simulink subsystem "Day6_Scenario_1"  (R2024a)
settings: Solver=VariableStepAuto  StartTime=0.0  StopTime=10.0  RelTol=1e-3
undefined symbols (not defined in the file): route1_waypoint, route2_waypoint, route3_waypoint
libraries: CarMaker4SL x15
settings Model: Creator=junhyung.cha  LastModifiedBy=User

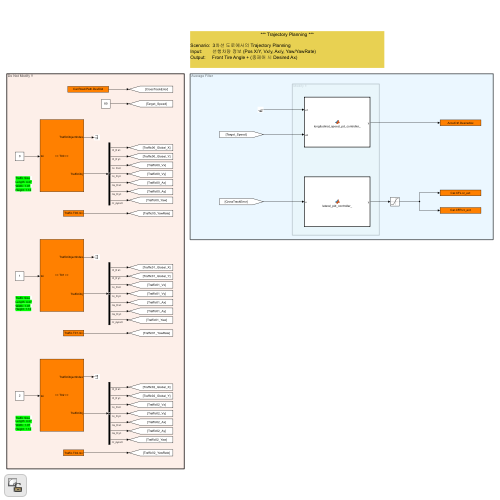
[thumbnail: Simulink's stored preview of the top-level diagram]
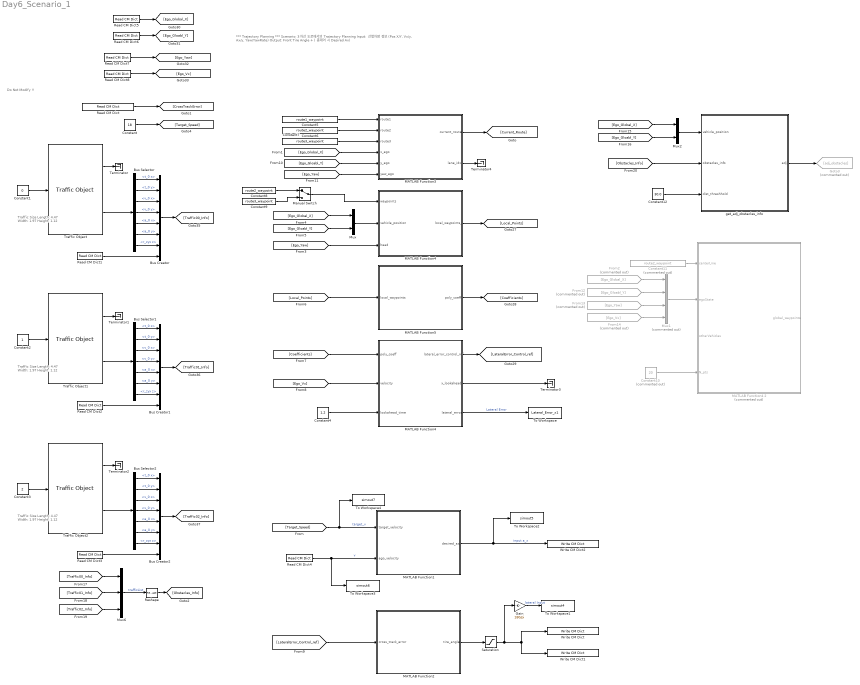
== system Day6_Scenario_1 ==
  note: Do Not Modify !!
  note: Traffic Size
      | Length: 4.47
      | Width: 1.97
      | Height: 1.12
  note: Traffic Size
      | Length: 4.47
      | Width: 1.97
      | Height: 1.12
  note: Traffic Size
      | Length: 4.47
      | Width: 1.97
      | Height: 1.12
  note: *** Trajectory Planning ***
      |
      | Scenario: 3차선 도로에서의 Trajectory Planning
      | Input: 선행차량 정보 (Pos X/Y, Vx/y, Ax/y, Yaw/YawRate)
      | Output: Front Tire Angle + (종제어 시 Desired Ax)
  Bus Creator : BusCreator  Inputs=8
  Bus Creator1 : BusCreator  Inputs=8
  Bus Creator2 : BusCreator  Inputs=8
  Bus Selector : BusSelector  OutputSignals=t_0 x,t_0 y,v_0 x,v_0 y,a_0 x,a_0 y,r_zyx z
  Bus Selector1 : BusSelector  OutputSignals=t_0 x,t_0 y,v_0 x,v_0 y,a_0 x,a_0 y,r_zyx z
  Bus Selector2 : BusSelector  OutputSignals=t_0 x,t_0 y,v_0 x,v_0 y,a_0 x,a_0 y,r_zyx z
  Constant : Constant  Value=18
  Constant1 : Constant  Value=0
  Constant10 : Constant  Commented=on  Value=20
  Constant11 : Constant  Commented=on  Value=route2_waypoint  SampleTime=-1
  Constant12 : Constant  Value=30.0
  Constant2 : Constant
  Constant3 : Constant  Value=2
  Constant4 : Constant  Value=1.2
  Constant5 : Constant  Value=route1_waypoint  SampleTime=-1
  Constant6 : Constant  Value=route2_waypoint  SampleTime=-1
  Constant7 : Constant  Value=route3_waypoint
  Constant8 : Constant  Value=route2_waypoint  SampleTime=-1
  Constant9 : Constant  Value=route3_waypoint
  From12 : From  Commented=on  GotoTag=Ego_Gloabl_Y
  From13 : From  Commented=on  GotoTag=Ego_Yaw
  From14 : From  Commented=on  GotoTag=Ego_Vx
  From2 : From  Commented=on  GotoTag=Ego_Global_X
  Gain : Gain  Gain=180/pi
  Goto3 : Goto  Commented=on  GotoTag=adj_obstacles
  MATLAB Function1 : MATLAB Function  TreatAsAtomicUnit=on
  MATLAB Function2 : MATLAB Function  TreatAsAtomicUnit=on
  MATLAB Function3 : MATLAB Function  TreatAsAtomicUnit=on
  MATLAB Function4 : MATLAB Function  TreatAsAtomicUnit=on
  "MATLAB Function4 " : MATLAB Function  TreatAsAtomicUnit=on
  MATLAB Function4 2 : MATLAB Function  Commented=on  TreatAsAtomicUnit=on
  MATLAB Function5 : MATLAB Function  TreatAsAtomicUnit=on
  Manual Switch : ManualSwitch  varsize=on
  Mux : Mux  Inputs=2
  Mux1 : Mux  Commented=on
  Mux2 : Mux  Inputs=2
  Mux6 : Mux  Inputs=3
  Read CM Dict : CarMaker4SL/Read CM Dict  xname=Car.Road.Path.DevDist  xsync=off  xstime=Inherited
  Read CM Dict1 : CarMaker4SL/Read CM Dict  xname=Traffic.T00.rzv  xsync=off  xstime=Inherited
  Read CM Dict2 : CarMaker4SL/Read CM Dict  xname=Traffic.T01.rzv  xsync=off  xstime=Inherited
  Read CM Dict3 : CarMaker4SL/Read CM Dict  xname=Traffic.T02.rzv  xsync=off  xstime=Inherited
  Read CM Dict4 : CarMaker4SL/Read CM Dict  xname=Car.v  xsync=off  xstime=Inherited
  Read CM Dict5 : CarMaker4SL/Read CM Dict  xname=Car.Fr1.tx  xsync=off  xstime=Inherited
  Read CM Dict6 : CarMaker4SL/Read CM Dict  xname=Car.Fr1.ty  xsync=off  xstime=Inherited
  Read CM Dict7 : CarMaker4SL/Read CM Dict  xname=Car.Fr1.rz  xsync=off  xstime=Inherited
  Read CM Dict8 : CarMaker4SL/Read CM Dict  xname=Car.v  xsync=off  xstime=Inherited
  Reshape : Reshape  OutputDimensionality=Customize  OutputDimensions=[3, 8]
  Saturation : Saturate  UpperLimit=2  LowerLimit=-2
  Terminator{,1..4} (5 alike) : Terminator
  To Workspace : ToWorkspace  VariableName=Lateral_Error_x1  SaveFormat=Timeseries  SampleTime=-1
  To Workspace1 : ToWorkspace  VariableName=simout4  SaveFormat=Timeseries  SampleTime=-1
  To Workspace2 : ToWorkspace  VariableName=simout5  SaveFormat=Timeseries  SampleTime=-1
  To Workspace3 : ToWorkspace  VariableName=simout6  SaveFormat=Timeseries  SampleTime=-1
  To Workspace4 : ToWorkspace  VariableName=simout7  SaveFormat=Timeseries  SampleTime=-1
  Traffic Object : CarMaker4SL/Traffic Object  xname=T00  ximode=Traffic Id  xstime=Inherited
      settings: SourceProductName=CarMaker4SL
  Traffic Object1 : CarMaker4SL/Traffic Object  xname=T01  ximode=Traffic Id  xstime=Inherited
      settings: SourceProductName=CarMaker4SL
  Traffic Object2 : CarMaker4SL/Traffic Object  xname=T02  ximode=Traffic Id  xstime=Inherited
      settings: SourceProductName=CarMaker4SL
  Write CM Dict : CarMaker4SL/Write CM Dict  xname=Car.CFL.rz_ext  xsync=off
  Write CM Dict1 : CarMaker4SL/Write CM Dict  xname=Car.CFR.rz_ext  xsync=off
  Write CM Dict2 : CarMaker4SL/Write CM Dict  xname=AccelCtrl.DesiredAx  xsync=off
  get_adj_obstacles_info : MATLAB Function  TreatAsAtomicUnit=on
  wires:
  Saturation/1 -> Write CM Dict1/1, Write CM Dict/1, Gain/1
  Constant1/1 -> Traffic Object/1
  MATLAB Function2/1(tire_angle) -> Saturation/1
  MATLAB Function1/1(desired_ax) -> Write CM Dict2/1, To Workspace2/1  "input a_x"
  [LateralError_Control_ref] -> MATLAB Function2/1(cross_track_error)
  Read CM Dict/1 -> [CrossTrackError]
  Constant/1 -> [Target_Speed]
  Bus Selector/4 -> Bus Creator/4  "<v_0 y>"
  Traffic Object/1 -> Terminator/1
  Bus Selector/3 -> Bus Creator/3  "<v_0 x>"
  Traffic Object/2 -> Bus Selector/1
  Bus Selector/1 -> Bus Creator/1  "<t_0 x>"
  Bus Selector/2 -> Bus Creator/2  "<t_0 y>"
  Read CM Dict1/1 -> Bus Creator/8
  Bus Selector/5 -> Bus Creator/5  "<a_0 x>"
  Bus Selector/6 -> Bus Creator/6  "<a_0 y>"
  Bus Selector/7 -> Bus Creator/7  "<r_zyx z>"
  Read CM Dict2/1 -> Bus Creator1/8
  Bus Selector1/1 -> Bus Creator1/1  "<t_0 x>"
  Bus Selector1/5 -> Bus Creator1/5  "<a_0 x>"
  Bus Selector1/6 -> Bus Creator1/6  "<a_0 y>"
  Bus Selector1/7 -> Bus Creator1/7  "<r_zyx z>"
  Traffic Object1/1 -> Terminator1/1
  Bus Selector1/4 -> Bus Creator1/4  "<v_0 y>"
  Constant2/1 -> Traffic Object1/1
  Bus Selector1/3 -> Bus Creator1/3  "<v_0 x>"
  Bus Selector1/2 -> Bus Creator1/2  "<t_0 y>"
  Bus Selector2/3 -> Bus Creator2/3  "<v_0 x>"
  Bus Selector2/2 -> Bus Creator2/2  "<t_0 y>"
  Bus Selector2/1 -> Bus Creator2/1  "<t_0 x>"
  Bus Selector2/6 -> Bus Creator2/6  "<a_0 y>"
  Constant3/1 -> Traffic Object2/1
  Traffic Object2/1 -> Terminator2/1
  Bus Selector2/7 -> Bus Creator2/7  "<r_zyx z>"
  Bus Selector2/5 -> Bus Creator2/5  "<a_0 x>"
  Read CM Dict3/1 -> Bus Creator2/8
  Bus Selector2/4 -> Bus Creator2/4  "<v_0 y>"
  [Target_Speed] -> MATLAB Function1/1(target_velocity), To Workspace4/1  "target_v"
  Read CM Dict4/1 -> MATLAB Function1/2(ego_velocity), To Workspace3/1  "v"
  [Ego_Gloabl_Y] -> Mux/2
  [Ego_Yaw] -> "MATLAB Function4 "/3(head)
  "MATLAB Function4 "/1(local_waypoints_) -> [Local_Points]
  Mux/1 -> "MATLAB Function4 "/2(vehicle_position)
  [Ego_Global_X] -> Mux/1
  MATLAB Function4/3(lateral_error) -> To Workspace/1  "Lateral Error"
  Constant4/1 -> MATLAB Function4/3(lookahead_time)
  MATLAB Function4/2(x_lookahead) -> Terminator3/1
  [Local_Points] -> MATLAB Function5/1(local_waypoints)
  MATLAB Function4/1(lateral_error_control_ref) -> [LateralError_Control_ref]
  MATLAB Function5/1(poly_coeff) -> [Coefficients]
  [Coefficients] -> MATLAB Function4/1(poly_coeff)
  [Ego_Vx] -> MATLAB Function4/2(velocity)
  [Ego_Global_X] -> MATLAB Function3/4(x_ego)
  [Ego_Gloabl_Y] -> MATLAB Function3/5(y_ego)
  [Ego_Yaw] -> MATLAB Function3/6(yaw_ego)
  MATLAB Function3/1(current_route) -> [Current_Route]
  Constant5/1 -> MATLAB Function3/1(route1)
  Constant6/1 -> MATLAB Function3/2(route2)
  Constant7/1 -> MATLAB Function3/3(route3)
  Read CM Dict5/1 -> [Ego_Global_X]
  Read CM Dict6/1 -> [Ego_Gloabl_Y]
  Read CM Dict8/1 -> [Ego_Vx]
  Read CM Dict7/1 -> [Ego_Yaw]
  Gain/1 -> To Workspace1/1  "lateral Input"
  Constant8/1 -> Manual Switch/1
  Constant9/1 -> Manual Switch/2
  Manual Switch/1 -> "MATLAB Function4 "/1(waypoints)
  Traffic Object1/2 -> Bus Selector1/1
  Traffic Object2/2 -> Bus Selector2/1
  Constant10/1 -> MATLAB Function4 2/4(N_pts)
  Constant11/1 -> MATLAB Function4 2/1(centerLine)
  From12/1 -> Mux1/2
  From2/1 -> Mux1/1
  From13/1 -> Mux1/3
  From14/1 -> Mux1/4
  Mux1/1 -> MATLAB Function4 2/2(egoState)
  [Ego_Gloabl_Y] -> Mux2/2
  [Ego_Global_X] -> Mux2/1
  Mux2/1 -> get_adj_obstacles_info/1(vehicle_position)
  Bus Creator/1 -> [Traffic00_Info]
  Bus Creator1/1 -> [Traffic01_Info]
  Bus Creator2/1 -> [Traffic02_Info]
  [Traffic00_Info] -> Mux6/1
  [Traffic01_Info] -> Mux6/2
  [Traffic02_Info] -> Mux6/3
  Mux6/1 -> Reshape/1  "trafficList"
  MATLAB Function3/2(lane_idx) -> Terminator4/1
  get_adj_obstacles_info/1(adj) -> Goto3/1
  Reshape/1 -> [Obstacles_Info]
  Constant12/1 -> get_adj_obstacles_info/3(dist_threshhold)
  [Obstacles_Info] -> get_adj_obstacles_info/2(obstacles_info)

== matlab function Day6_Scenario_1/MATLAB Function1 ==
  settings: updateMethod=DISCRETE  sampleTime=0.1
  data: target_velocity input; desired_ax output; ego_velocity input
function desired_ax = longitudinal_speed_pi_controller_(target_velocity, ego_velocity)
    desired_ax = longitudinal_speed_pi_controller_mfile(target_velocity, ego_velocity);
end


function desired_ax = longitudinal_speed_pi_controller_mfile(target_velocity, ego_velocity)
     
    persistent error_sum
    dt = 0.1;
    
    error = target_velocity - ego_velocity;

    if isempty(error_sum)
        error_sum = 0;
    else
        error_sum = error_sum + error * dt;
    end

    Kp = 0.215;
    Ki = 0.001;

    P_term = Kp*error;
    I_term = Ki*error_sum;
    
    desired_ax = (P_term + I_term);

end

== matlab function Day6_Scenario_1/MATLAB Function2 ==
  settings: updateMethod=DISCRETE  sampleTime=0.05
  data: cross_track_error input; tire_angle output
function tire_angle = lateral_pid_controller_(cross_track_error)
    tire_angle = lateral_pid_controller_mfile(cross_track_error);
end

function tire_angle = lateral_pid_controller_mfile(cross_track_error)
    persistent error_prev error_sum
    % error = average_filter_mfile(cross_track_error);
    error = cross_track_error;
    
    dt = 0.05;

    if isempty(error_prev)
        error_prev = error;
    end

    if isempty(error_sum)
        error_sum = 0;
    else
        error_sum = error_sum + error * dt;
    end

    Kp = 0.03;
    Ki = 0.001;
    Kd = 0.005;
  
    P_term = Kp*error;
    I_term = Ki*error_sum;
    D_term = Kd*(error - error_prev) / dt;
    
    tire_angle = (P_term + I_term + D_term);
    error_prev = error;
end

== matlab function Day6_Scenario_1/MATLAB Function3 ==
  settings: sampleTime=0.1
  data: route1 input; current_route output; route2 input; route3 input; x_ego input; y_ego input; yaw_ego input; lane_idx output
    function [current_route, lane_idx] = current_lane_identifier(route1, route2, route3, x_ego, y_ego, yaw_ego)
    
        w_theta = 0.5;
        
        routes = {route1, route2, route3};
        scores = zeros(3,1);
        
        for k = 1:3
            route = routes{k};
            
            % projection distance + lane direction
            [d_proj, theta_lane] = proj_distance(route, x_ego, y_ego);
            
            % heading error
            diff = yaw_ego - theta_lane;
            heading_err = abs(atan2(sin(diff), cos(diff)));
            
            scores(k) = d_proj + w_theta * heading_err;
        end
        
        [~, lane_idx] = min(scores);
        
        current_route = routes{lane_idx};
        %disp(lane_idx)
    end


function [d_min, theta_lane] = proj_distance(route, x, y)
    N = size(route,1);
    p = [x; y];
    
    d_min = 1e9;
    theta_lane = 0;
    
    for i = 1:N-1
        p1 = route(i,:)';
        p2 = route(i+1,:)';
        
        v = p2 - p1;
        u = p - p1;
        
        denom = v' * v;
        if denom < 1e-9
            continue;
        end
        
        % projection factor
        t = (u' * v) / denom;
        t = max(0, min(1, t));   % clamp to segment
        
        % projected point
        p_proj = p1 + t * v;
        
        % distance
        d = norm(p - p_proj);
        
        if d < d_min
            d_min = d;
            theta_lane = atan2(v(2), v(1));  % segment 방향
        end
    end
end

== matlab function Day6_Scenario_1/MATLAB Function4  ==
  settings: updateMethod=DISCRETE  sampleTime=0.05
  data: waypoints input; local_waypoints_ output size=[20 2]; vehicle_position input; head input
function local_waypoints_ = global_to_local_waypoints(waypoints, vehicle_position, head)
    local_waypoints_ = global_to_local_waypoints_mfile(waypoints, vehicle_position, head);
end

function local_waypoints_ = global_to_local_waypoints_mfile(waypoints, vehicle_position, head)

    num_waypoint = 20;
    vehicle_position = vehicle_position(:)';

    dx = waypoints(:,1) - vehicle_position(1);
    dy = waypoints(:,2) - vehicle_position(2);
    dist = dx.^2 + dy.^2;

    isNotForward = (dx*cos(head) + dy*sin(head)) < 0;
    dist(isNotForward) = inf;

    [~, idx_start] = min(dist);

    idx_end = idx_start + num_waypoint - 1;
    idx_end = min(idx_end, size(waypoints,1));
    selected = waypoints(idx_start:idx_end, :);

    L = size(selected,1);
    if L < num_waypoint
        selected = [selected; repmat(selected(end,:), num_waypoint-L, 1)];
    end

    R_inv = [ cos(head),  sin(head);
             -sin(head),  cos(head) ];

    delta = bsxfun(@minus, selected, vehicle_position);
    local_waypoints_ = (R_inv * delta')';

end

== matlab function Day6_Scenario_1/MATLAB Function4 ==
  settings: updateMethod=DISCRETE  sampleTime=0.05
  data: lateral_error_control_ref output; x_lookahead output; poly_coeff input; lateral_error output; velocity input; lookahead_time input
function [lateral_error_control_ref, x_lookahead, lateral_error] = compute_lateral_error(poly_coeff, velocity, lookahead_time)
    [lateral_error_control_ref, x_lookahead, lateral_error] = compute_lateral_error_mfile(poly_coeff, velocity, lookahead_time);
end


function [lateral_error_control_ref, x_lookahead, lateral_error] = compute_lateral_error_mfile(poly_coeff, velocity, lookahead_time)

    x_lookahead = velocity * lookahead_time;
    degree = length(poly_coeff) - 1;

    y_ref = 0;
    for i = 0:degree
        y_ref = y_ref + poly_coeff(i+1) * x_lookahead^i;
    end

    lateral_error_control_ref = y_ref;
    lateral_error = poly_coeff(1);
    
end

== matlab function Day6_Scenario_1/MATLAB Function5 ==
  settings: updateMethod=DISCRETE  sampleTime=0.05
  data: local_waypoints input; poly_coeff output
function poly_coeff = fit_polynomial_to_waypoints(local_waypoints)
    poly_coeff = fit_polynomial_to_waypoints_mfile(local_waypoints);
end

function poly_coeff = fit_polynomial_to_waypoints_mfile(local_waypoints)
    
    num_degree = 3;
    N = size(local_waypoints, 1);

    x = local_waypoints(:,1);
    b = local_waypoints(:,2);

    A = zeros(N, num_degree+1);
    for i = 0:num_degree
        A(:, i+1) = x.^i;
    end
    
    poly_coeff = pinv(A) * b;
    
end

== matlab function Day6_Scenario_1/get_adj_obstacles_info ==
  settings: updateMethod=DISCRETE  sampleTime=0.05
  data: vehicle_position input; obstacles_info input [3..10]; adj output; dist_threshhold input
function adj = get_adj_obstacles_info(vehicle_position, obstacles_info, dist_threshhold)

    % vehicle_position : [x, y] (EGO global position)
    % obstacles_info   : Nx matrix or struct (each obstacle row = one vehicle)
    %                    columns assumed: [X, Y, Vx, Vy, Ax, Ay, Yaw, Yawrate]
    % dist_thresh      : scalar (e.g., 50 meters)
    
    disp('--------')
    disp(obstacles_info);
    disp('--------')
    disp('Vehicle_position')
    disp(vehicle_position);
    disp('--------')
    ego_x = vehicle_position(1);
    ego_y = vehicle_position(2);

    X = obstacles_info(:,1);
    Y = obstacles_info(:,2);

    % 거리 계산
    dx = X - ego_x;
    dy = Y - ego_y;
    dist = dx.^2 + dy.^2;

    % threshold 안에 있는 인덱스
    idx = dist < dist_threshhold^2;
    disp(idx);

    % 필터링된 장애물 정보
    adj = obstacles_info(idx, :);
    
    if ~isempty(adj)
        disp('-----')
        disp(adj(1));
        disp(adj(1, :));
    end
end

== matlab function Day6_Scenario_1/MATLAB Function4 2 ==
  settings: updateMethod=DISCRETE  sampleTime=0.05
  data: centerLine input; egoState input; global_waypoints output size=[20 2]; otherVehicles input; N_pts input
function global_waypoints  = planOptimalTrajectory(centerLine, egoState, otherVehicles, N_pts)
    % centerLine: Nx2 [X, Y]
    % egoState: [x, y, yaw, v, a]
    % otherVehicles: Mx6 [x, y, vx, vy, ax, ay] (M은 가변)
    % N_pts: 출력할 trajectory 점 개수
    % 출력: x_traj, y_traj - N_pts x 1 trajectory
    
    % coder.varsize 지정 (Simulink/Codegen 호환)
    coder.varsize('otherVehicles', [20, 6]);
    
    laneWidth = 3.5;
    dList = [-laneWidth/2.0, 0.0, laneWidth/2.0];
    targetSpeed = 20.0;
    TimeList = [1.0, 1.5, 2.0];

    [si, di, yaw_ref] = globalToFrenet(centerLine, egoState(1:2), egoState(3));
    v = egoState(4);
    a = egoState(5);
    si_dot = v * cos(egoState(3) - yaw_ref);
    si_ddot = a * cos(egoState(3) - yaw_ref);
    di_dot = v * sin(egoState(3) - yaw_ref);
    di_ddot = a * sin(egoState(3) - yaw_ref);

    sf_dot = targetSpeed;
    
    trajSet = {};
    costs = [];

    for i = 1:3
        df = dList(i);
        for j = 1:3
            T = TimeList(j);

            coeff_d = quinticPoly(di, di_dot, di_ddot, df, 0, 0, T);
            coeff_s = quarticPoly(si, si_dot, si_ddot, sf_dot, 0, T);

            [s_traj, d_traj, s_dot, d_dot, s_ddot, d_ddot, s_jerk, d_jerk] = sampleTrajectory(coeff_s, coeff_d, T, N_pts);

            [x_traj_tmp, y_traj_tmp] = frenetToGlobal(s_traj, d_traj, centerLine);
            kappa = computeCurvature(x_traj_tmp, y_traj_tmp);

            if ~checkConstraints(s_traj, d_traj, s_dot, d_dot, s_ddot, d_ddot, kappa, otherVehicles, centerLine)
                continue;
            end

            cost = computeCost(s_jerk, d_jerk, T, di, s_dot(end), df, targetSpeed);

            trajSet{end+1} = [x_traj_tmp, y_traj_tmp];
            costs(end+1) = cost;

        end
    end

    if isempty(costs)
        x_traj = zeros(N_pts, 1);
        y_traj = zeros(N_pts, 1);
    else
        [~, idx] = min(costs);
        x_traj = trajSet{idx}(:,1);
        y_traj = trajSet{idx}(:,2);
    end

    global_waypoints = [x_traj, y_traj];

end

function coeff = quinticPoly(xi, vi, ai, xf, vf, af, T)
    A = [T^3,    T^4,     T^5;
         3*T^2,  4*T^3,   5*T^4;
         6*T,    12*T^2,  20*T^3];

    b = [xf - (xi + vi*T + 0.5*ai*T^2);
         vf - (vi + ai*T);
         af - ai];

    x = A \ b;

    coeff = [xi, vi, 0.5*ai, x(1), x(2), x(3)];
end

function coeff = quarticPoly(xi, vi, ai, vf, af, T)
    A = [3*T^2,    4*T^3;
         6*T,     12*T^2];

    b = [vf - (vi + ai*T);
         af - ai];

    x = A \ b;

    coeff = [xi, vi, 0.5*ai, x(1), x(2)];
end

function [s, d, heading] = globalToFrenet(centerLine, x, y)
    min_dist = inf;
    closest_idx = 1;

    % 가장 가까운 segment 찾기
    for i = 1:size(centerLine,1)-1
        p1 = centerLine(i,:)';
        p2 = centerLine(i+1,:)';
        proj = projectionOnSegment([x; y], p1, p2);
        dist = norm([x; y] - proj);
        if dist < min_dist
            min_dist = dist;
            closest_idx = i;
            proj_point = proj;
            segment_vec = p2 - p1;
        end
    end

    % cumulative s 계산
    s = 0;
    for i = 1:closest_idx-1
        s = s + norm(centerLine(i+1,:) - centerLine(i,:));
    end
    s = s + norm(proj_point' - centerLine(closest_idx,:));

    % d 계산
    heading = atan2(segment_vec(2), segment_vec(1));
    normal = [-sin(heading); cos(heading)]; % 왼쪽 수직 방향
    d = dot(([x; y] - proj_point), normal);
end


function proj = projectionOnSegment(p, p1, p2)
    % p: 2x1, p1, p2: 2x1
    v = p2 - p1;
    t = dot(p - p1, v) / dot(v, v);
    t = max(0, min(1, t));
    proj = p1 + t * v;
end

function [s_traj, d_traj, s_dot, d_dot, s_ddot, d_ddot, s_jerk, d_jerk] = sampleTrajectory(coeff_s, coeff_d, T, N_pts)
    t_vec = linspace(0, T, N_pts)';

    % s(t), s_dot(t), s_ddot(t), s_jerk(t)
    s_traj = polyval(flip(coeff_s), t_vec);
    s_dot = polyval(polyder(flip(coeff_s)), t_vec);
    s_ddot = polyval(polyder(polyder(flip(coeff_s))), t_vec);
    s_jerk = polyval(polyder(polyder(polyder(flip(coeff_s)))), t_vec);

    % d(t), d_dot(t), d_ddot(t), d_jerk(t)
    d_traj = polyval(flip(coeff_d), t_vec);
    d_dot = polyval(polyder(flip(coeff_d)), t_vec);
    d_ddot = polyval(polyder(polyder(flip(coeff_d))), t_vec);
    d_jerk = polyval(polyder(polyder(polyder(flip(coeff_d)))), t_vec);
end

function [x_traj, y_traj] = frenetToGlobal(s_traj, d_traj, centerLine)
    % s_traj, d_traj : N x 1 (frenet trajectory)
    % centerLine : M x 2 (global waypoints)
    % x_traj, y_traj : N x 1 (global trajectory)
    
    
    N = length(s_traj);
    x_traj = zeros(N, 1);
    y_traj = zeros(N, 1);
    
    
    % 사전 cumulative s 계산
    s_map = zeros(size(centerLine,1),1);
    for i = 2:length(centerLine)
        ds = norm(centerLine(i,:) - centerLine(i-1,:));
        s_map(i) = s_map(i-1) + ds;
    end
    
    
    for i = 1:N
        s = s_traj(i);
        d = d_traj(i);
        
        
        % s 기준 위치 찾기
        idx = find(s_map >= s, 1);
        if isempty(idx) || idx == 1
            idx = 2;
        end
    
        s0 = s_map(idx-1);
        s1 = s_map(idx);
        p0 = centerLine(idx-1,:);
        p1 = centerLine(idx,:);
        
        
        heading = atan2(p1(2) - p0(2), p1(1) - p0(1));
        ratio = (s - s0) / (s1 - s0);
        px = p0(1) + ratio * (p1(1) - p0(1));
        py = p0(2) + ratio * (p1(2) - p0(2));
        
    
        normal = [-sin(heading), cos(heading)];
        x_traj(i) = px + d * normal(1);
        y_traj(i) = py + d * normal(2);
    end

end

function valid = checkConstraints(s_traj, d_traj, s_dot, d_dot, s_ddot, d_ddot, kappa, otherVehicles, centerLine)
    V_MAX     = 50.0;
    A_MAX     = 2.0;
    KAPPA_MAX = 2.0;
    COLL_DIST = 1.5;
    % 속도 제약
    v = s_dot.^2 + d_dot.^2;
    if any(v > V_MAX^2)
        valid = false;
        return;
    end
    
    % 가속도 제약
    acc = s_ddot.^2 + d_ddot.^2;
    if any(acc > A_MAX^2)
        valid = false;
        return;
    end

    % 곡률 제약
    if any(abs(kappa) > KAPPA_MAX)
        valid = false;
        return;
    end

    % 충돌 확인
    [x_traj, y_traj] = frenetToGlobal(s_traj, d_traj, centerLine);
    for i = 1:size(otherVehicles,1)
        veh_x = otherVehicles(i,1);
        veh_y = otherVehicles(i,2);

        dist2 = (x_traj - veh_x).^2 + (y_traj - veh_y).^2;
        if any(dist2 < COLL_DIST^2) % 충돌 반경 0.25m
            valid = false;
            return;
        end
    end

    valid = true;
end

function cost = computeCost(s_jerk, d_jerk, T, di, sf_dot, df, TARGET_SPEED)
    % 가중치
    K_J = 0.1;
    K_T = 0.1;
    K_D = 1.0;
    K_V = 1.0;
    K_LAT = 1.0;
    K_LON = 1.0;
    
    J_lat = sum(d_jerk.^2);
    J_lon = sum(s_jerk.^2);
    
    d_diff = (df - di)^2;
    v_diff = (TARGET_SPEED - sf_dot)^2;
    
    c_lat = K_J * J_lat + K_T * T + K_D * d_diff;
    c_lon = K_J * J_lon + K_T * T + K_V * v_diff;
    
    cost = K_LAT * c_lat + K_LON * c_lon;
end

function kappa = computeCurvature(x, y)
    dx = gradient(x);
    dy = gradient(y);
    ddx = gradient(dx);
    ddy = gradient(dy);
    
    kappa = (dx .* ddy - dy .* ddx) ./ ((dx.^2 + dy.^2).^(3/2));
end
